simulink model "kei_ledblink2_sl"  (R2020b)
settings: Solver=FixedStepDiscrete  StartTime=0.0  StopTime=10.0  RelTol=1e-3
libraries: arduino_io_lib x3
settings Model: Creator=kei55  LastModifiedBy=kei55

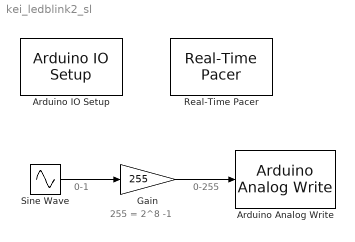
== system kei_ledblink2_sl ==
  note: 0-255
  note: 0-1
  note: 255 = 2^8 -1
  Arduino Analog Write : arduino_io_lib/Arduino Analog Write  arduinoVar=Temporary arduino variable: Arduino1  arduinoPin=11  T=1/50
  Arduino IO Setup : arduino_io_lib/Arduino IO Setup  Priority=3  arduinoVar=Temporary arduino variable: Arduino1  workspaceVarName=a  comPort=COM3
  Gain : Gain  Gain=255
  Real-Time Pacer : arduino_io_lib/Real-Time Pacer  simTimePerRealTime=1
  Sine Wave : Sin  SineType=Sample based  Amplitude=0.5  Bias=0.5  Samples=50  SampleTime=1/50
  wires:
  Sine Wave/1 -> Gain/1
  Gain/1 -> Arduino Analog Write/1
